simulink model "TEST_IPM_2_0"  (R2019b)
settings: configuration reference "Configuration" (kept outside this file)
PreLoadFcn:
  | RTWConfigurationCB('preloadfcn', bdroot);
values from neighbouring files (symbols this model uses):
  MParamFbase = 200.0    [TEST_IPM_LIB.sldd]
  MParamIbase = 360.0    [TEST_IPM_LIB.sldd]
  MParamLd = 8.0E-5    [TEST_IPM_LIB.sldd]
  MParamLq = 0.00028    [TEST_IPM_LIB.sldd]
  MParamRs = 0.014    [TEST_IPM_LIB.sldd]
  PWM_TPBRD_HALF = 5000.0    [TEST_IPM_LIB.sldd]
  Ts_10kHz = 0.0001    [TEST_IPM_LIB.sldd]
  Ts_1kHz = 0.001    [TEST_IPM_LIB.sldd]
undefined symbols (not defined in the file or in its folder): DiscIntNeverNeededParam, Down, GPTRIP1SEL, GPTRIP2SEL, TZ1, TZ2, Up
libraries: c280xlib x24, c2837xDlib x18, dsparch4 x11, c2802xlib x10, powerlib_meascontrol x9, dspstat3 x2, c2000lib x1, c2806xlib x1, idelinklib_common x1
(part 4 of 6)

== system TEST_IPM_2_0/INT/MAX5742/Subsystem3 ==
  function : TriggerPort  TriggerType=function-call  VariantControl=Variant
  Add1 : Sum
  Add3 : Sum  Commented=on
  Constant1 : Constant  Value=hex2dec('3000')  OutDataTypeStr=uint16  SampleTime=-1
  Constant6 : Constant  Commented=on  Value=hex2dec('3000')  OutDataTypeStr=uint16  SampleTime=-1
  Data Store Read : DataStoreRead  DataStoreName=Udc_FBK
  Data Store Read21 : DataStoreRead  Commented=on  DataStoreName=N_NOFILTER
  Gain1 : Gain  Commented=on  Gain=1/3000*4095
  Gain2 : Gain  Gain=1/80*4095
  SPI Transmit1 : c280xlib/SPI Transmit  SPISelect=SPI_B  ClockPolarity=Rising_edge  ClockPhase=No_delay  SPIModule=uint32(0)  Mode=Master  BusSpeed=uint32(1000000)  FirstBitToTransfer=Most significant bit (MSB)  ClockMode=0  BlockFunction=Write  EnableRegisterAddress=on  RegisterAddress=0  OutputDataType=int8  OutputDataLength=1  BlockingMode=off  DataBits=16  UseCustomSSPin=Provided by the SPI peripheral  ActiveLowSSPin=Active low  Pin=0
      settings: SourceProductName=Embedded Coder Support Package for Texas Instruments C2000 Processors  SourceProductBaseCode=TIC2000
  SPI Transmit3 : c280xlib/SPI Transmit  Commented=on  SPISelect=SPI_B  ClockPolarity=Rising_edge  ClockPhase=No_delay  SPIModule=uint32(0)  Mode=Master  BusSpeed=uint32(1000000)  FirstBitToTransfer=Most significant bit (MSB)  ClockMode=0  BlockFunction=Write  EnableRegisterAddress=on  RegisterAddress=0  OutputDataType=int8  OutputDataLength=1  BlockingMode=off  DataBits=16  UseCustomSSPin=Provided by the SPI peripheral  ActiveLowSSPin=Active low  Pin=0
      settings: SourceProductName=Embedded Coder Support Package for Texas Instruments C2000 Processors  SourceProductBaseCode=TIC2000
  Saturation1 : Saturate  UpperLimit=4095  LowerLimit=0  OutDataTypeStr=uint16
  Saturation3 : Saturate  Commented=on  UpperLimit=4095  LowerLimit=0  OutDataTypeStr=uint16
  Terminator1 : Terminator
  Terminator3 : Terminator  Commented=on
  wires:
  SPI Transmit3/1 -> Terminator3/1
  Constant6/1 -> Add3/2
  Gain1/1 -> Saturation3/1
  Saturation3/1 -> Add3/1
  Add3/1 -> SPI Transmit3/1
  Data Store Read21/1 -> Gain1/1
  Data Store Read/1 -> Gain2/1
  Add1/1 -> SPI Transmit1/1
  Saturation1/1 -> Add1/1
  Gain2/1 -> Saturation1/1
  Constant1/1 -> Add1/2
  SPI Transmit1/1 -> Terminator1/1

== system TEST_IPM_2_0/INT/MAX5742/Subsystem4 ==
  function : TriggerPort  TriggerType=function-call  VariantControl=Variant
  Add2 : Sum
  Constant1 : Constant  Value=hex2dec('0000')  OutDataTypeStr=uint16  SampleTime=-1
  Constant2 : Constant  Priority=102  Value=1024  OutDataTypeStr=Inherit: Inherit via back propagation  SampleTime=-1
  SPI Transmit : c280xlib/SPI Transmit  SPISelect=SPI_B  ClockPolarity=Rising_edge  ClockPhase=No_delay  SPIModule=uint32(0)  Mode=Master  BusSpeed=uint32(1000000)  FirstBitToTransfer=Most significant bit (MSB)  ClockMode=0  BlockFunction=Write  EnableRegisterAddress=on  RegisterAddress=0  OutputDataType=int8  OutputDataLength=1  BlockingMode=off  DataBits=16  UseCustomSSPin=Provided by the SPI peripheral  ActiveLowSSPin=Active low  Pin=0
      settings: SourceProductName=Embedded Coder Support Package for Texas Instruments C2000 Processors  SourceProductBaseCode=TIC2000
  Saturation : Saturate  UpperLimit=4095  LowerLimit=0  OutDataTypeStr=uint16
  Terminator : Terminator
  wires:
  Constant1/1 -> Add2/2
  SPI Transmit/1 -> Terminator/1
  Saturation/1 -> Add2/1
  Constant2/1 -> Saturation/1
  Add2/1 -> SPI Transmit/1

== system TEST_IPM_2_0/INT/MAX5742/Subsystem5 ==
  function : TriggerPort  TriggerType=function-call  VariantControl=Variant
  Add1 : Sum
  Constant1 : Constant  Priority=107  Value=2048  OutDataTypeStr=Inherit: Inherit via back propagation  SampleTime=-1
  Constant2 : Constant  Value=hex2dec('1000')  OutDataTypeStr=uint16  SampleTime=-1
  SPI Transmit1 : c280xlib/SPI Transmit  SPISelect=SPI_B  ClockPolarity=Rising_edge  ClockPhase=No_delay  SPIModule=uint32(0)  Mode=Master  BusSpeed=uint32(1000000)  FirstBitToTransfer=Most significant bit (MSB)  ClockMode=0  BlockFunction=Write  EnableRegisterAddress=on  RegisterAddress=0  OutputDataType=int8  OutputDataLength=1  BlockingMode=off  DataBits=16  UseCustomSSPin=Provided by the SPI peripheral  ActiveLowSSPin=Active low  Pin=0
      settings: SourceProductName=Embedded Coder Support Package for Texas Instruments C2000 Processors  SourceProductBaseCode=TIC2000
  Saturation1 : Saturate  UpperLimit=4095  LowerLimit=0  OutDataTypeStr=uint16
  Terminator1 : Terminator
  wires:
  Saturation1/1 -> Add1/1
  Add1/1 -> SPI Transmit1/1
  SPI Transmit1/1 -> Terminator1/1
  Constant2/1 -> Add1/2
  Constant1/1 -> Saturation1/1

== system TEST_IPM_2_0/INT/MAX5742/Subsystem6 ==
  function : TriggerPort  TriggerType=function-call  VariantControl=Variant
  Add4 : Sum
  Constant1 : Constant  Priority=112  Value=3072  OutDataTypeStr=Inherit: Inherit via back propagation  SampleTime=-1
  Constant5 : Constant  Value=hex2dec('2000')  OutDataTypeStr=uint16  SampleTime=-1
  SPI Transmit2 : c280xlib/SPI Transmit  SPISelect=SPI_B  ClockPolarity=Rising_edge  ClockPhase=No_delay  SPIModule=uint32(0)  Mode=Master  BusSpeed=uint32(1000000)  FirstBitToTransfer=Most significant bit (MSB)  ClockMode=0  BlockFunction=Write  EnableRegisterAddress=on  RegisterAddress=0  OutputDataType=int8  OutputDataLength=1  BlockingMode=off  DataBits=16  UseCustomSSPin=Provided by the SPI peripheral  ActiveLowSSPin=Active low  Pin=0
      settings: SourceProductName=Embedded Coder Support Package for Texas Instruments C2000 Processors  SourceProductBaseCode=TIC2000
  Saturation2 : Saturate  UpperLimit=4095  LowerLimit=0  OutDataTypeStr=uint16
  Terminator2 : Terminator
  wires:
  Constant5/1 -> Add4/2
  Saturation2/1 -> Add4/1
  Add4/1 -> SPI Transmit2/1
  SPI Transmit2/1 -> Terminator2/1
  Constant1/1 -> Saturation2/1

== system TEST_IPM_2_0/INT/MAX5742/Subsystem7 ==
  function : TriggerPort  TriggerType=function-call  VariantControl=Variant
  Add3 : Sum
  Constant6 : Constant  Value=hex2dec('3000')  OutDataTypeStr=uint16  SampleTime=-1
  Data Store Read : DataStoreRead  DataStoreName=UDCPROTECT
  SPI Transmit3 : c280xlib/SPI Transmit  SPISelect=SPI_B  ClockPolarity=Rising_edge  ClockPhase=No_delay  SPIModule=uint32(0)  Mode=Master  BusSpeed=uint32(1000000)  FirstBitToTransfer=Most significant bit (MSB)  ClockMode=0  BlockFunction=Write  EnableRegisterAddress=on  RegisterAddress=0  OutputDataType=int8  OutputDataLength=1  BlockingMode=off  DataBits=16  UseCustomSSPin=Provided by the SPI peripheral  ActiveLowSSPin=Active low  Pin=0
      settings: SourceProductName=Embedded Coder Support Package for Texas Instruments C2000 Processors  SourceProductBaseCode=TIC2000
  Saturation3 : Saturate  UpperLimit=4095  LowerLimit=0  OutDataTypeStr=uint16
  Terminator3 : Terminator
  wires:
  SPI Transmit3/1 -> Terminator3/1
  Constant6/1 -> Add3/2
  Data Store Read/1 -> Saturation3/1
  Saturation3/1 -> Add3/1
  Add3/1 -> SPI Transmit3/1

== system TEST_IPM_2_0/INT/Motor Control/Adjusting Mode ==
  Action Port : ActionPort  ActionPortLabel=case [ 0 ]:

== system TEST_IPM_2_0/INT/Motor Control/Clark Transformation ==
  U : Inport
  V : Inport  Port=2
  W : Inport  Port=3
  Add : Sum  Inputs=+--
  Add1 : Sum  Inputs=+-
  Gain : Gain  Gain=0.5
  Gain1 : Gain  Gain=0.5
  Gain2 : Gain  Gain=2/3
  Gain3 : Gain  Gain=2/3*0.86602540
  Alpha : Outport
  Beta : Outport  Port=2
  wires:
  V/1 -> Add1/1, Gain/1
  Gain/1 -> Add/2
  W/1 -> Add1/2, Gain1/1
  Gain1/1 -> Add/3
  U/1 -> Add/1
  Add/1 -> Gain2/1
  Gain2/1 -> Alpha/1
  Add1/1 -> Gain3/1
  Gain3/1 -> Beta/1

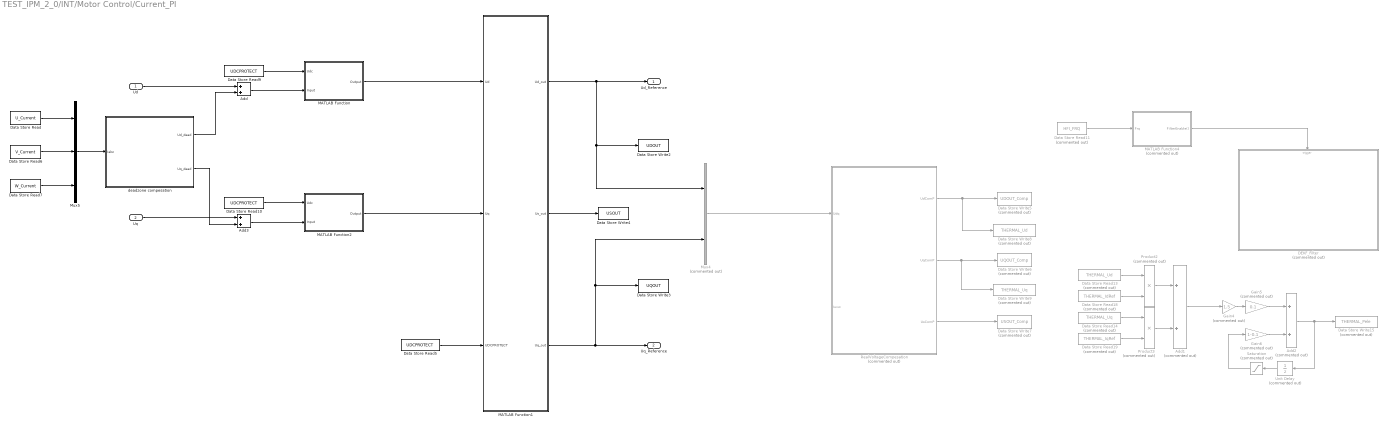
== system TEST_IPM_2_0/INT/Motor Control/Current_PI ==
  Ud : Inport
  Uq : Inport  Port=2
  Add : Sum
  Add1 : Sum  Commented=on
  Add2 : Sum  Commented=on
  Add3 : Sum
  DEKF_Filter : Subsystem  Commented=on  TreatAsAtomicUnit=on
  Data Store Read : DataStoreRead  DataStoreName=U_Current
  Data Store Read10 : DataStoreRead  DataStoreName=UDCPROTECT
  Data Store Read11 : DataStoreRead  Commented=on  DataStoreName=HFI_FRQ
  Data Store Read13 : DataStoreRead  Commented=on  DataStoreName=THERMAL_Ud
  Data Store Read14 : DataStoreRead  Commented=on  DataStoreName=THERMAL_Uq
  Data Store Read18 : DataStoreRead  Commented=on  DataStoreName=THERMAL_IdRef
  Data Store Read19 : DataStoreRead  Commented=on  DataStoreName=THERMAL_IqRef
  Data Store Read5 : DataStoreRead  DataStoreName=UDCPROTECT
  Data Store Read6 : DataStoreRead  DataStoreName=V_Current
  Data Store Read7 : DataStoreRead  DataStoreName=W_Current
  Data Store Read9 : DataStoreRead  DataStoreName=UDCPROTECT
  Data Store Write15 : DataStoreWrite  Commented=on  DataStoreName=THERMAL_Pele
  Data Store Write2 : DataStoreWrite  DataStoreName=UDOUT
  Data Store Write3 : DataStoreWrite  DataStoreName=UQOUT
  Data Store Write4 : DataStoreWrite  DataStoreName=USOUT
  Data Store Write5 : DataStoreWrite  Commented=on  DataStoreName=UDOUT_Comp
  Data Store Write6 : DataStoreWrite  Commented=on  DataStoreName=UQOUT_Comp
  Data Store Write7 : DataStoreWrite  Commented=on  DataStoreName=USOUT_Comp
  Data Store Write8 : DataStoreWrite  Commented=on  DataStoreName=THERMAL_Ud
  Data Store Write9 : DataStoreWrite  Commented=on  DataStoreName=THERMAL_Uq
  Gain4 : Gain  Commented=on  Gain=1.5
  Gain5 : Gain  Commented=on  Gain=0.1
  Gain6 : Gain  Commented=on  Gain=1-0.1
  MATLAB Function : MATLAB Function  TreatAsAtomicUnit=on
  MATLAB Function1 : MATLAB Function  TreatAsAtomicUnit=on
  MATLAB Function2 : MATLAB Function  TreatAsAtomicUnit=on
  MATLAB Function4 : MATLAB Function  Commented=on  TreatAsAtomicUnit=on
  Mux4 : Mux  Commented=on  Inputs=2
  Mux5 : Mux  Inputs=3
  Product2 : Product  Commented=on
  Product3 : Product  Commented=on
  "RealVoltageCompesation " : Subsystem  Commented=on  TreatAsAtomicUnit=on
  Saturation : Saturate  Commented=on  UpperLimit=100e3  LowerLimit=-100e3
  Unit Delay : UnitDelay  Commented=on  SampleTime=-1  HasFrameUpgradeWarning=on
  deadzone compesation : Subsystem
  Ud_Reference : Outport
  Uq_Reference : Outport  Port=2
  wires:
  MATLAB Function1/1(Ud_out) -> Ud_Reference/1, Data Store Write2/1, Mux4/1
  MATLAB Function1/3(Uq_out) -> Uq_Reference/1, Mux4/2, Data Store Write3/1
  MATLAB Function1/2(Us_out) -> Data Store Write4/1
  Data Store Read5/1 -> MATLAB Function1/3(UDCPROTECT)
  Mux4/1 -> "RealVoltageCompesation "/1(Udq)
  Data Store Read/1 -> Mux5/1
  Data Store Read6/1 -> Mux5/2
  Data Store Read7/1 -> Mux5/3
  Data Store Read9/1 -> MATLAB Function/1(Udc)
  Data Store Read10/1 -> MATLAB Function2/1(Udc)
  MATLAB Function/1(Output) -> MATLAB Function1/1(Ud)
  MATLAB Function2/1(Output) -> MATLAB Function1/2(Uq)
  "RealVoltageCompesation "/2(UqComP) -> Data Store Write9/1, Data Store Write6/1
  "RealVoltageCompesation "/3(UsComP) -> Data Store Write7/1
  "RealVoltageCompesation "/1(UdComP) -> Data Store Write8/1, Data Store Write5/1
  MATLAB Function4/1(FilterEnable()) -> DEKF_Filter/Trigger
  Data Store Read11/1 -> MATLAB Function4/1(Frq)
  Data Store Read13/1 -> Product2/1
  Data Store Read18/1 -> Product2/2
  Data Store Read14/1 -> Product3/1
  Data Store Read19/1 -> Product3/2
  Product2/1 -> Add1/1
  Product3/1 -> Add1/2
  Add1/1 -> Gain4/1
  Gain4/1 -> Gain5/1
  Add2/1 -> Unit Delay/1, Data Store Write15/1
  Unit Delay/1 -> Saturation/1
  Gain5/1 -> Add2/1
  Gain6/1 -> Add2/2
  Saturation/1 -> Gain6/1
  Add/1 -> MATLAB Function/2(Input)
  Ud/1 -> Add/1
  Add3/1 -> MATLAB Function2/2(Input)
  Uq/1 -> Add3/1
  deadzone compesation/1(Ud_dead) -> Add/2
  deadzone compesation/2(Uq_dead) -> Add3/2
  Mux5/1 -> deadzone compesation/1(Iabc)

== system TEST_IPM_2_0/INT/Motor Control/Error ==
  Action Port : ActionPort  ActionPortLabel=default:
  Constant : Constant  OutDataTypeStr=Inherit: Inherit via back propagation  SampleTime=-1
  Constant1 : Constant  Value=0  OutDataTypeStr=Inherit: Inherit via back propagation  SampleTime=-1
  Data Store Write1 : DataStoreWrite  DataStoreName=PROTECT
  Data Store Write2 : DataStoreWrite  DataStoreName=STOP
  wires:
  Constant/1 -> Data Store Write2/1
  Constant1/1 -> Data Store Write1/1

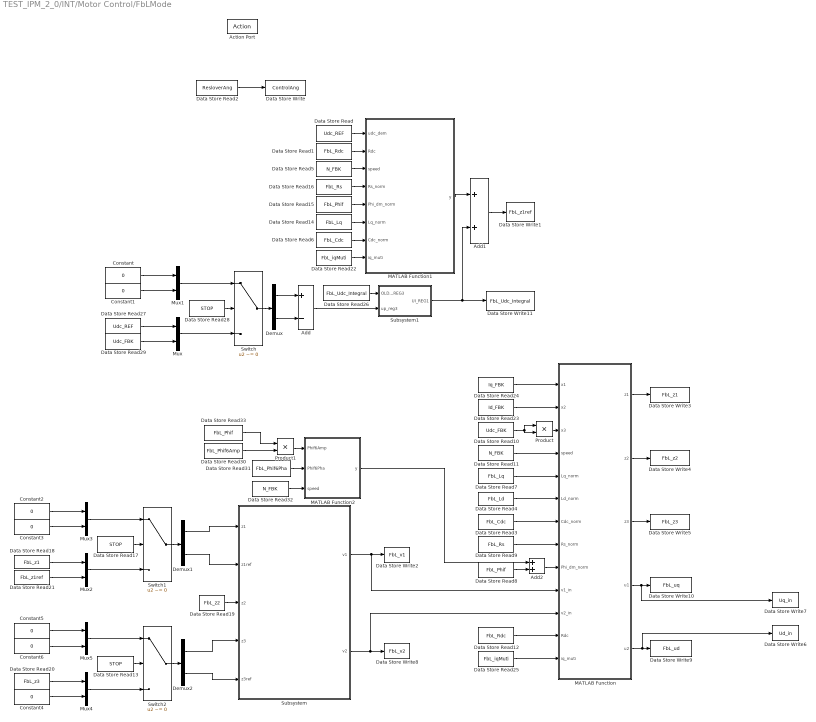
== system TEST_IPM_2_0/INT/Motor Control/FbLMode ==
  Action Port : ActionPort  ActionPortLabel=case [ 6 ]:
  Add : Sum  Inputs=+-
  Add1 : Sum
  Add2 : Sum
  Constant{,1..3,5..6} (6 alike) : Constant  Value=0  OutDataTypeStr=single  SampleTime=-1
  Constant4 : Constant  Value=0  OutDataTypeStr=single
  Data Store Read : DataStoreRead  DataStoreName=Udc_REF
  Data Store Read1 : DataStoreRead  DataStoreName=FbL_Rdc
  Data Store Read10 : DataStoreRead  DataStoreName=Udc_FBK
  Data Store Read11 : DataStoreRead  DataStoreName=N_FBK
  Data Store Read12 : DataStoreRead  DataStoreName=FbL_Rdc
  Data Store Read13 : DataStoreRead  DataStoreName=STOP
  Data Store Read14 : DataStoreRead  DataStoreName=FbL_Lq
  Data Store Read15 : DataStoreRead  DataStoreName=FbL_Phif
  Data Store Read16 : DataStoreRead  DataStoreName=FbL_Rs
  Data Store Read17 : DataStoreRead  DataStoreName=STOP
  Data Store Read18 : DataStoreRead  DataStoreName=FbL_z1
  Data Store Read19 : DataStoreRead  DataStoreName=FbL_z2
  Data Store Read2 : DataStoreRead  DataStoreName=ResloverAng
  Data Store Read20 : DataStoreRead  DataStoreName=FbL_z3
  Data Store Read21 : DataStoreRead  DataStoreName=FbL_z1ref
  Data Store Read22 : DataStoreRead  DataStoreName=FbL_iqMuti
  Data Store Read23 : DataStoreRead  DataStoreName=Id_FBK
  Data Store Read24 : DataStoreRead  DataStoreName=Iq_FBK
  Data Store Read25 : DataStoreRead  DataStoreName=FbL_iqMuti
  Data Store Read26 : DataStoreRead  DataStoreName=FbL_Udc_Integral
  Data Store Read27 : DataStoreRead  DataStoreName=Udc_REF
  Data Store Read28 : DataStoreRead  DataStoreName=STOP
  Data Store Read29 : DataStoreRead  DataStoreName=Udc_FBK
  Data Store Read3 : DataStoreRead  DataStoreName=FbL_Cdc
  Data Store Read30 : DataStoreRead  DataStoreName=FbL_Phif6Amp
  Data Store Read31 : DataStoreRead  DataStoreName=FbL_Phif6Pha
  Data Store Read32 : DataStoreRead  DataStoreName=N_FBK
  Data Store Read33 : DataStoreRead  DataStoreName=FbL_Phif
  Data Store Read4 : DataStoreRead  DataStoreName=FbL_Ld
  Data Store Read5 : DataStoreRead  DataStoreName=N_FBK
  Data Store Read6 : DataStoreRead  DataStoreName=FbL_Cdc
  Data Store Read7 : DataStoreRead  DataStoreName=FbL_Lq
  Data Store Read8 : DataStoreRead  DataStoreName=FbL_Phif
  Data Store Read9 : DataStoreRead  DataStoreName=FbL_Rs
  Data Store Write : DataStoreWrite  DataStoreName=ControlAng
  Data Store Write1 : DataStoreWrite  DataStoreName=FbL_z1ref
  Data Store Write10 : DataStoreWrite  DataStoreName=FbL_uq
  Data Store Write11 : DataStoreWrite  DataStoreName=FbL_Udc_Integral
  Data Store Write2 : DataStoreWrite  DataStoreName=FbL_v1
  Data Store Write3 : DataStoreWrite  DataStoreName=FbL_z1
  Data Store Write4 : DataStoreWrite  DataStoreName=FbL_z2
  Data Store Write5 : DataStoreWrite  DataStoreName=FbL_z3
  Data Store Write6 : DataStoreWrite  DataStoreName=Ud_in
  Data Store Write7 : DataStoreWrite  DataStoreName=Uq_in
  Data Store Write8 : DataStoreWrite  DataStoreName=FbL_v2
  Data Store Write9 : DataStoreWrite  DataStoreName=FbL_ud
  Demux : Demux  Outputs=2
  Demux1 : Demux  Outputs=2
  Demux2 : Demux  Outputs=2
  MATLAB Function : MATLAB Function  TreatAsAtomicUnit=on
  MATLAB Function1 : MATLAB Function  TreatAsAtomicUnit=on
  MATLAB Function2 : MATLAB Function  TreatAsAtomicUnit=on
  Mux{,1..5} (6 alike) : Mux  Inputs=2
  Product : Product
  Product1 : Product
  Subsystem : Subsystem
  Subsystem1 : Subsystem
  Switch : Switch  Criteria=u2 ~= 0
  Switch1 : Switch  Criteria=u2 ~= 0
  Switch2 : Switch  Criteria=u2 ~= 0
  wires:
  Data Store Read2/1 -> Data Store Write/1
  Data Store Read1/1 -> MATLAB Function1/2(Rdc)
  Data Store Read/1 -> MATLAB Function1/1(udc_dem)
  Data Store Read5/1 -> MATLAB Function1/3(speed)
  Data Store Read14/1 -> MATLAB Function1/6(Lq_norm)
  Data Store Read6/1 -> MATLAB Function1/7(Cdc_norm)
  Data Store Read16/1 -> MATLAB Function1/4(Rs_norm)
  Data Store Read15/1 -> MATLAB Function1/5(Phi_dm_norm)
  Subsystem1/1(UI_REG1) -> Data Store Write11/1, Add1/2
  Add/1 -> Subsystem1/2(up_reg3)
  MATLAB Function1/1(y) -> Add1/1
  Data Store Read19/1 -> Subsystem/3(z2)
  Add1/1 -> Data Store Write1/1
  Subsystem/1(v1) -> MATLAB Function/10(v1_in), Data Store Write2/1
  Subsystem/2(v2) -> Data Store Write8/1, MATLAB Function/11(v2_in)
  Data Store Read26/1 -> Subsystem1/1(OLD_UI_REG3)
  Data Store Read29/1 -> Mux/2
  Demux/2 -> Add/2
  Data Store Read27/1 -> Mux/1
  Demux/1 -> Add/1
  Constant/1 -> Mux1/1
  Constant1/1 -> Mux1/2
  Mux1/1 -> Switch/1
  Switch/1 -> Demux/1
  Data Store Read28/1 -> Switch/2
  Mux/1 -> Switch/3
  Data Store Read17/1 -> Switch1/2
  Constant3/1 -> Mux3/2
  Mux2/1 -> Switch1/3
  Constant2/1 -> Mux3/1
  Demux1/1 -> Subsystem/1(z1)
  Switch1/1 -> Demux1/1
  Demux1/2 -> Subsystem/2(z1ref)
  Mux3/1 -> Switch1/1
  Data Store Read18/1 -> Mux2/1
  Data Store Read21/1 -> Mux2/2
  Mux5/1 -> Switch2/1
  Switch2/1 -> Demux2/1
  Constant5/1 -> Mux5/1
  Mux4/1 -> Switch2/3
  Constant6/1 -> Mux5/2
  Data Store Read13/1 -> Switch2/2
  Data Store Read20/1 -> Mux4/1
  Constant4/1 -> Mux4/2
  Demux2/1 -> Subsystem/4(z3)
  Demux2/2 -> Subsystem/5(z3ref)
  Data Store Read7/1 -> MATLAB Function/5(Lq_norm)
  Data Store Read10/1 -> Product/2, Product/1
  Data Store Read3/1 -> MATLAB Function/7(Cdc_norm)
  MATLAB Function/5(u2) -> Data Store Write6/1, Data Store Write9/1
  Data Store Read24/1 -> MATLAB Function/1(x1)
  Data Store Read4/1 -> MATLAB Function/6(Ld_norm)
  MATLAB Function/1(z1) -> Data Store Write3/1
  Data Store Read9/1 -> MATLAB Function/8(Rs_norm)
  MATLAB Function/3(z3) -> Data Store Write5/1
  MATLAB Function/4(u1) -> Data Store Write7/1, Data Store Write10/1
  Data Store Read11/1 -> MATLAB Function/4(speed)
  MATLAB Function/2(z2) -> Data Store Write4/1
  Data Store Read12/1 -> MATLAB Function/12(Rdc)
  Product/1 -> MATLAB Function/3(x3)
  Data Store Read23/1 -> MATLAB Function/2(x2)
  Data Store Read22/1 -> MATLAB Function1/8(iq_muti)
  Data Store Read25/1 -> MATLAB Function/13(iq_muti)
  Data Store Read31/1 -> MATLAB Function2/2(Phif6Pha)
  Data Store Read32/1 -> MATLAB Function2/3(speed)
  Add2/1 -> MATLAB Function/9(Phi_dm_norm)
  Data Store Read8/1 -> Add2/2
  MATLAB Function2/1(y) -> Add2/1
  Product1/1 -> MATLAB Function2/1(Phif6Amp)
  Data Store Read30/1 -> Product1/2
  Data Store Read33/1 -> Product1/1

== system TEST_IPM_2_0/INT/Motor Control/IF ==
  Action Port : ActionPort  ActionPortLabel=case [ 2 ]:
  Data Store Read2 : DataStoreRead  DataStoreName=IF_F
  Data Store Read3 : DataStoreRead  DataStoreName=IF_F_Step
  Data Store Write : DataStoreWrite  DataStoreName=ControlAng
  Subsystem1 : Subsystem
  Subsystem2 : Subsystem
  wires:
  Data Store Read3/1 -> Subsystem1/2(Step)
  Data Store Read2/1 -> Subsystem1/1(TargetValue)
  Subsystem2/1(Ang) -> Data Store Write/1
  Subsystem1/1(RampOutput) -> Subsystem2/1(FRQ)

== system TEST_IPM_2_0/INT/Motor Control/Park Transformation ==
  Alpha : Inport
  Beta : Inport  Port=2
  theta : Inport  Port=3
  Add : Sum
  Add1 : Sum  Inputs=+-
  Product{,1..3} (4 alike) : Product
  Sin : Trigonometry  OutputSignalType=real
  Sin1 : Trigonometry  Operator=cos  OutputSignalType=real
  D : Outport
  Q : Outport  Port=2
  wires:
  Product/1 -> Add/1
  Sin/1 -> Product3/2, Product1/2
  Product1/1 -> Add/2
  Add1/1 -> Q/1
  Sin1/1 -> Product2/2, Product/2
  Product2/1 -> Add1/1
  Alpha/1 -> Product3/1, Product/1
  Beta/1 -> Product2/1, Product1/1
  Product3/1 -> Add1/2
  Add/1 -> D/1
  theta/1 -> Sin/1, Sin1/1

== system TEST_IPM_2_0/INT/Motor Control/SVPWM ==
  note: 由于矿车控制器ePWMxA是下管，B是上管，所以add变成了++
  Ud_Reference : Inport
  Uq_Reference : Inport  Port=2
  Angle : Inport  Port=3
  Add : Sum
  Constant1 : Constant  Value=PWM_TPBRD_HALF  OutDataTypeStr=single  SampleTime=-1
  Data Store Read3 : DataStoreRead  DataStoreName=ControlMode
  Data Store Read4 : DataStoreRead  DataStoreName=N_FBK
  Data Store Read5 : DataStoreRead  DataStoreName=Udc_FBK
  Demux : Demux  Outputs=2
  Divide : Product  Inputs=*/
  Gain : Gain  Gain=1/sqrt(3)
  Gain1 : Gain  Gain=PWM_TPBRD_HALF  OutDataTypeStr=single  ParamDataTypeStr=Inherit: Same as input
  Gain2 : Gain  Gain=4/60*2*pi*Ts_10kHz*1.5
  Inverse Park Transformation : Subsystem
  MATLAB Function : MATLAB Function  TreatAsAtomicUnit=on
  MATLAB Function1 : MATLAB Function  TreatAsAtomicUnit=on
  Mux : Mux  Inputs=2
  Mux1 : Mux  Inputs=3
  Saturation : Saturate  UpperLimit=370  LowerLimit=10
  Sum1 : Sum  Inputs=|-+  OutDataTypeStr=uint16
  COMPARE : Outport
  wires:
  Inverse Park Transformation/1(Alpha) -> MATLAB Function/1(alpha)
  Inverse Park Transformation/2(Beta) -> MATLAB Function/2(beta)
  Mux1/1 -> Gain1/1
  Sum1/1 -> COMPARE/1
  Gain1/1 -> Sum1/1
  Constant1/1 -> Sum1/2
  MATLAB Function/3(tc) -> Mux1/3
  MATLAB Function/2(tb) -> Mux1/2
  MATLAB Function/1(ta) -> Mux1/1
  Ud_Reference/1 -> Mux/1
  Uq_Reference/1 -> Mux/2
  Mux/1 -> Divide/1
  Saturation/1 -> Divide/2
  Gain/1 -> Saturation/1
  Demux/1 -> Inverse Park Transformation/1(D)
  Demux/2 -> Inverse Park Transformation/2(Q)
  Divide/1 -> Demux/1
  Data Store Read5/1 -> Gain/1
  Data Store Read4/1 -> Gain2/1
  Angle/1 -> Add/1
  Gain2/1 -> Add/2
  Add/1 -> MATLAB Function1/1(theta_in)
  Data Store Read3/1 -> MATLAB Function1/2(controlmode)
  MATLAB Function1/1(theta_out) -> Inverse Park Transformation/3(theta)

== system TEST_IPM_2_0/INT/Motor Control/SpeedMode ==
  Action Port : ActionPort  ActionPortLabel=case [ 4 ]:
  Constant3 : Constant  Value=MParamFbase*2*pi*MParamLq*1.5  OutDataTypeStr=Inherit: Inherit via back propagation  SampleTime=-1
  Constant4 : Constant  Value=MParamFbase*2*pi*MParamRs*1.5  OutDataTypeStr=Inherit: Inherit via back propagation  SampleTime=-1
  Constant5 : Constant  Value=MParamFbase*2*pi*MParamLq*1.5  OutDataTypeStr=Inherit: Inherit via back propagation  SampleTime=-1
  Constant6 : Constant  Value=MParamFbase*2*pi*MParamRs*1.5  OutDataTypeStr=Inherit: Inherit via back propagation  SampleTime=-1
  Data Store Read{,4..6} (4 alike) : DataStoreRead  DataStoreName=PI_Multi
  Data Store Read1 : DataStoreRead  Commented=on  DataStoreName=FLAG_MTPA
  Data Store Read2 : DataStoreRead  DataStoreName=ResloverAng
  Data Store Read3 : DataStoreRead  Commented=on  DataStoreName=Iq_REF
  Data Store Write : DataStoreWrite  DataStoreName=ControlAng
  Data Store Write3 : DataStoreWrite  DataStoreName=Id_Ki
  Data Store Write4 : DataStoreWrite  DataStoreName=Id_Kp
  Data Store Write5 : DataStoreWrite  DataStoreName=Iq_Ki
  Data Store Write6 : DataStoreWrite  DataStoreName=Iq_Kp
  Function-Call Subsystem : Subsystem  TreatAsAtomicUnit=on
  MATLAB Function : MATLAB Function  TreatAsAtomicUnit=on
  MATLAB Function1 : MATLAB Function  Commented=on  TreatAsAtomicUnit=on
  Product{,1..3} (4 alike) : Product
  wires:
  Data Store Read2/1 -> Data Store Write/1
  MATLAB Function/1(Speed_PI()) -> Function-Call Subsystem/Trigger
  Data Store Read3/1 -> MATLAB Function1/2(IqDem)
  Data Store Read1/1 -> MATLAB Function1/1(Flag_MTPA)
  MATLAB Function1/1(Id_REF) -> ?
  Product/1 -> Data Store Write4/1
  Data Store Read/1 -> Product/2
  Constant3/1 -> Product/1
  Constant4/1 -> Product1/1
  Data Store Read4/1 -> Product1/2
  Product1/1 -> Data Store Write3/1
  Product3/1 -> Data Store Write5/1
  Data Store Read6/1 -> Product3/2
  Constant6/1 -> Product3/1
  Constant5/1 -> Product2/1
  Data Store Read5/1 -> Product2/2
  Product2/1 -> Data Store Write6/1

== system TEST_IPM_2_0/INT/Motor Control/Stop  ==
  Action Port : ActionPort  ActionPortLabel=case [ 5 ]:
  Constant3 : Constant  OutDataTypeStr=Inherit: Inherit via back propagation  SampleTime=-1
  Constant4 : Constant  Value=0  OutDataTypeStr=Inherit: Inherit via back propagation  SampleTime=-1
  Data Store Write3 : DataStoreWrite  DataStoreName=PROTECT
  Data Store Write4 : DataStoreWrite  DataStoreName=STOP
  wires:
  Constant3/1 -> Data Store Write4/1
  Constant4/1 -> Data Store Write3/1

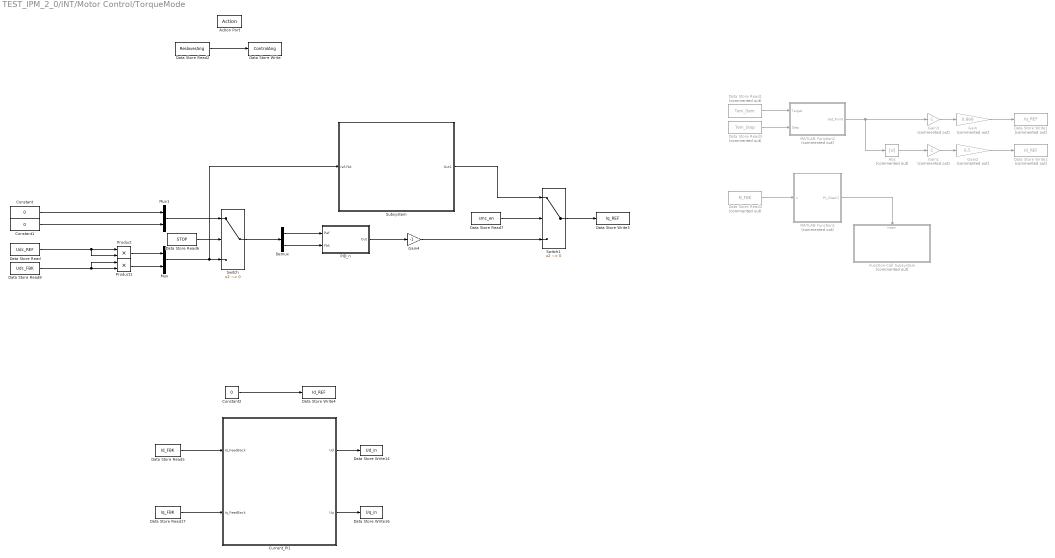
== system TEST_IPM_2_0/INT/Motor Control/TorqueMode ==
  Action Port : ActionPort  ActionPortLabel=case [ 3 ]:
  Abs : Abs  Commented=on
  Constant : Constant  Value=0  OutDataTypeStr=single  SampleTime=-1
  Constant1 : Constant  Value=0  OutDataTypeStr=single  SampleTime=-1
  Constant2 : Constant  Value=0  OutDataTypeStr=single
  Current_PI1 : Subsystem  TreatAsAtomicUnit=on
      settings: RTWSystemCode=Inline
  Data Store Read : DataStoreRead  DataStoreName=Udc_REF
  Data Store Read1 : DataStoreRead  Commented=on  DataStoreName=Tem_Dem
  Data Store Read17 : DataStoreRead  DataStoreName=Iq_FBK
  Data Store Read2 : DataStoreRead  DataStoreName=ResloverAng
  Data Store Read3 : DataStoreRead  Commented=on  DataStoreName=Tem_Step
  Data Store Read4 : DataStoreRead  Commented=on  DataStoreName=N_FBK
  Data Store Read5 : DataStoreRead  DataStoreName=Id_FBK
  Data Store Read6 : DataStoreRead  DataStoreName=STOP
  Data Store Read7 : DataStoreRead  DataStoreName=smc_en
  Data Store Read8 : DataStoreRead  DataStoreName=Udc_FBK
  Data Store Write : DataStoreWrite  DataStoreName=ControlAng
  Data Store Write1 : DataStoreWrite  Commented=on  DataStoreName=Iq_REF
  Data Store Write14 : DataStoreWrite  DataStoreName=Ud_in
  Data Store Write16 : DataStoreWrite  DataStoreName=Uq_in
  Data Store Write2 : DataStoreWrite  Commented=on  DataStoreName=Id_REF
  Data Store Write3 : DataStoreWrite  DataStoreName=Iq_REF
  Data Store Write4 : DataStoreWrite  DataStoreName=Id_REF
  Demux : Demux  Outputs=2
  Function-Call Subsystem : Subsystem  Commented=on  TreatAsAtomicUnit=on
  Gain : Gain  Commented=on  Gain=0.866
  Gain1 : Gain  Commented=on  Gain=-1  OutDataTypeStr=single
  Gain2 : Gain  Commented=on  Gain=0.5
  Gain3 : Gain  Commented=on  Gain=-1  OutDataTypeStr=single
  Gain4 : Gain  Gain=-1
  MATLAB Function1 : MATLAB Function  Commented=on  TreatAsAtomicUnit=on
  MATLAB Function2 : MATLAB Function  Commented=on  TreatAsAtomicUnit=on
  Mux : Mux  Inputs=2
  Mux1 : Mux  Inputs=2
  "PID_n " : Subsystem
  Product : Product
  Product1 : Product
  Subsystem : Subsystem
  Switch : Switch  Criteria=u2 ~= 0
  Switch1 : Switch  Criteria=u2 ~= 0
  wires:
  Data Store Read2/1 -> Data Store Write/1
  Data Store Read1/1 -> MATLAB Function2/1(Target)
  Data Store Read3/1 -> MATLAB Function2/2(Step)
  MATLAB Function2/1(Set_Point) -> Gain3/1, Abs/1
  Abs/1 -> Gain1/1
  Gain/1 -> Data Store Write1/1
  Gain1/1 -> Gain2/1
  Gain2/1 -> Data Store Write2/1
  Data Store Read4/1 -> MATLAB Function1/1(n)
  MATLAB Function1/1(PI_Clear()) -> Function-Call Subsystem/Trigger
  Gain3/1 -> Gain/1
  Demux/2 -> "PID_n "/2(Fbk)
  Mux/1 -> Subsystem/1(ref-fbk), Switch/3
  Mux1/1 -> Switch/1
  Constant/1 -> Mux1/1
  Switch/1 -> Demux/1
  Constant1/1 -> Mux1/2
  Demux/1 -> "PID_n "/1(Ref)
  Data Store Read6/1 -> Switch/2
  "PID_n "/1(Out) -> Gain4/1
  Constant2/1 -> Data Store Write4/1
  Current_PI1/2(Uq) -> Data Store Write16/1
  Current_PI1/1(Ud) -> Data Store Write14/1
  Data Store Read17/1 -> Current_PI1/2(Iq_FeedBack)
  Data Store Read5/1 -> Current_PI1/1(Id_FeedBack)
  Product/1 -> Mux/1
  Data Store Read/1 -> Product/2, Product/1
  Product1/1 -> Mux/2
  Data Store Read8/1 -> Product1/1, Product1/2
  Data Store Read7/1 -> Switch1/2
  Subsystem/1(Out1) -> Switch1/1
  Gain4/1 -> Switch1/3
  Switch1/1 -> Data Store Write3/1

== system TEST_IPM_2_0/INT/Motor Control/VF ==
  Action Port : ActionPort  ActionPortLabel=case [ 1 ]:
  Data Store Read : DataStoreRead  DataStoreName=VF_F
  Data Store Read2 : DataStoreRead  DataStoreName=VF_F_Step
  Data Store Write : DataStoreWrite  DataStoreName=ControlAng
  Subsystem1 : Subsystem
  Subsystem2 : Subsystem
  wires:
  Subsystem1/1(RampOutput) -> Subsystem2/1(FRQ)
  Subsystem2/1(Ang) -> Data Store Write/1
  Data Store Read/1 -> Subsystem1/1(TargetValue)
  Data Store Read2/1 -> Subsystem1/2(Step)

== system TEST_IPM_2_0/INT/Read Rotor Position/SpeedCal ==
  In1 : Inport
  function : TriggerPort  TriggerType=function-call  VariantControl=Variant
  "First Order Filter " : Subsystem
  MATLAB Function1 : MATLAB Function  TreatAsAtomicUnit=on
  Unit Delay : UnitDelay  SampleTime=-1  HasFrameUpgradeWarning=on
  Out1 : Outport
  wires:
  In1/1 -> Unit Delay/1, MATLAB Function1/1(theta)
  Unit Delay/1 -> MATLAB Function1/2(theta_old)
  MATLAB Function1/1(speed) -> "First Order Filter "/1(input)
  "First Order Filter "/1("output ") -> Out1/1

== system TEST_IPM_2_0/INT/ePWM/If Action Subsystem ==
  Action Port : ActionPort  ActionPortLabel=if(u1 == 1)
  Constant : Constant  Value=0  OutDataTypeStr=single  SampleTime=-1
  Data Store Write : DataStoreWrite  DataStoreName=N_Integral
  Data Store Write1 : DataStoreWrite  DataStoreName=Iq_Integral
  Data Store Write10 : DataStoreWrite  DataStoreName=FbL_z1_Integral
  Data Store Write12 : DataStoreWrite  DataStoreName=FbL_Udc_Integral
  Data Store Write2 : DataStoreWrite  DataStoreName=Id_Integral
  Data Store Write3 : DataStoreWrite  DataStoreName=Udc_Integral
  Data Store Write4 : DataStoreWrite  DataStoreName=smc_x1_integral
  Data Store Write5 : DataStoreWrite  DataStoreName=smc_e1_integral
  Data Store Write6 : DataStoreWrite  DataStoreName=smc_z1_integral
  Data Store Write7 : DataStoreWrite  DataStoreName=FbL_smc_integral
  Data Store Write9 : DataStoreWrite  DataStoreName=FbL_z3_Integral
  wires:
  Constant/1 -> Data Store Write3/1, Data Store Write10/1, Data Store Write7/1, Data Store Write6/1, Data Store Write5/1, Data Store Write4/1, Data Store Write12/1, Data Store Write9/1, Data Store Write1/1, Data Store Write2/1, Data Store Write/1

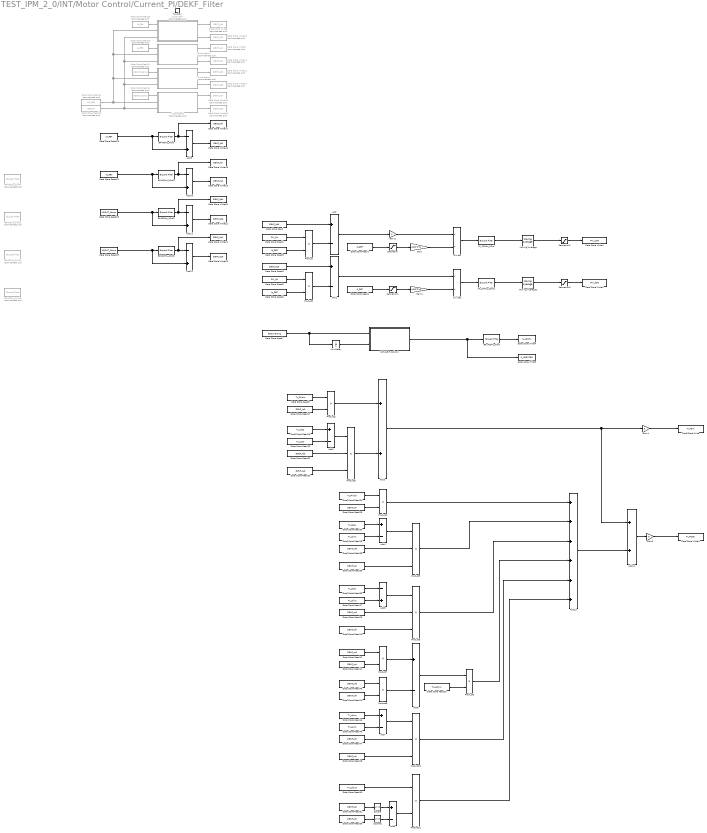
== system TEST_IPM_2_0/INT/Motor Control/Current_PI/DEKF_Filter ==
  function : TriggerPort  TriggerType=function-call  VariantControl=Variant  StatesWhenEnabling=reset
  Add{,1..2,4,6..8} (7 alike) : Sum  Inputs=+-
  Add{5,9..12} (5 alike) : Sum  Inputs=-+
  Add13 : Sum  Inputs=++++++
  Add14 : Sum
  Add3 : Sum
  BP400Hz_2Ord{1..4} (4 alike) : dsparch4/Biquad Filter  Tag=BlockMethodSubSystem  Commented=on  FilterSource=Dialog parameters  CoeffSource=Specify via dialog  FilterObject=BQF  IIRFiltStruct=Direct form II  BiQuadCoeffs=[1 0 -1 1 -1.92510858784585936 0.987511929907313402]  ScaleValues=[0.00624403504634327925;1]  IC=0  ICnum=0  ICden=0  a0Flag=Warning  optimizeScaleValues=on  ScaleValueMode=Specify via input port (g)  InputProcessing=Columns as channels (frame based)  roundingMode=Floor  overflowMode=off  scaleValueFracLength=14  denProdOutputFracLength=30  denAccumFracLength=30  secondMemoryFracLength=15
      settings: SourceProductName=DSP System Toolbox
  BP400Hz_4Ord{,1..3} (4 alike) : dsparch4/Biquad Filter  Tag=BlockMethodSubSystem  FilterSource=Dialog parameters  CoeffSource=Specify via dialog  FilterObject=BQF  IIRFiltStruct=Direct form II  BiQuadCoeffs=[1 0 -1 1 -1.93173306238314613 0.995528700328886185;1 0 -1 1 -1.93401211185528576 0.995605245274684303]  ScaleValues=[0.00313463184767947276;0.00313463184767947276;1]  IC=0  ICnum=0  ICden=0  a0Flag=Warning  optimizeScaleValues=on  ScaleValueMode=Specify via input port (g)  InputProcessing=Columns as channels (frame based)  roundingMode=Floor  overflowMode=off  scaleValueFracLength=14  denProdOutputFracLength=30  denAccumFracLength=30  secondMemoryFracLength=15
      settings: SourceProductName=DSP System Toolbox
  BP_400Hz_4Ord : dsparch4/Biquad Filter  Tag=BlockMethodSubSystem  FilterSource=Dialog parameters  CoeffSource=Specify via dialog  FilterObject=BQF  IIRFiltStruct=Direct form II  BiQuadCoeffs=[1 0 -1 1 -1.93173306238314613 0.995528700328886185;1 0 -1 1 -1.93401211185528576 0.995605245274684303]  ScaleValues=[0.00313463184767947276;0.00313463184767947276;1]  IC=0  ICnum=0  ICden=0  a0Flag=Warning  optimizeScaleValues=on  ScaleValueMode=Specify via input port (g)  InputProcessing=Columns as channels (frame based)  roundingMode=Floor  overflowMode=off  scaleValueFracLength=14  denProdOutputFracLength=30  denAccumFracLength=30  secondMemoryFracLength=15
      settings: SourceProductName=DSP System Toolbox
  Data Store Read : DataStoreRead  DataStoreName=DEKF_Ud0
  Data Store Read1 : DataStoreRead  DataStoreName=N_REF
  Data Store Read10 : DataStoreRead  DataStoreName=Tr_Lqap
  Data Store Read11 : DataStoreRead  Commented=on  DataStoreName=UDOUT_Comp
  Data Store Read12 : DataStoreRead  Commented=on  DataStoreName=HFI_FRQ
  Data Store Read13 : DataStoreRead  Commented=on  DataStoreName=DEKF_K
  Data Store Read14 : DataStoreRead  Commented=on  DataStoreName=UQOUT_Comp
  Data Store Read15 : DataStoreRead  DataStoreName=Tr_Lqinc
  Data Store Read16 : DataStoreRead  DataStoreName=Tr_Ldap
  Data Store Read17 : DataStoreRead  DataStoreName=Tr_Ldinc
  Data Store Read18 : DataStoreRead  DataStoreName=Id_FBK
  Data Store Read19 : DataStoreRead  DataStoreName=UDOUT_Comp
  Data Store Read2 : DataStoreRead  DataStoreName=Phi_Rs
  Data Store Read20 : DataStoreRead  DataStoreName=Tr_Ldqinc
  Data Store Read23 : DataStoreRead  DataStoreName=UQOUT_Comp
  Data Store Read24 : DataStoreRead  DataStoreName=Iq_FBK
  Data Store Read25 : DataStoreRead  Commented=on  DataStoreName=Id_FBK
  Data Store Read26 : DataStoreRead  Commented=on  DataStoreName=Iq_FBK
  Data Store Read{27,29,32,42} (4 alike) : DataStoreRead  DataStoreName=DEKF_Iq0
  Data Store Read{28,36,41,48,51} (5 alike) : DataStoreRead  DataStoreName=DEKF_Iqh
  Data Store Read3 : DataStoreRead  DataStoreName=DEKF_Uq0
  Data Store Read31 : DataStoreRead  DataStoreName=DEKF_Id0
  Data Store Read33 : DataStoreRead  DataStoreName=Tr_Ldap
  Data Store Read34 : DataStoreRead  DataStoreName=Tr_Phidm
  Data Store Read35 : DataStoreRead  DataStoreName=DEKF_Id0
  Data Store Read39 : DataStoreRead  DataStoreName=Tr_Lqap
  Data Store Read4 : DataStoreRead  DataStoreName=N_REF
  Data Store Read{40,44,47,50} (4 alike) : DataStoreRead  DataStoreName=DEKF_Idh
  Data Store Read43 : DataStoreRead  DataStoreName=DEKF_Id0
  Data Store Read45 : DataStoreRead  DataStoreName=Tr_Lqinc
  Data Store Read46 : DataStoreRead  DataStoreName=Tr_Ldinc
  Data Store Read49 : DataStoreRead  DataStoreName=Tr_Ldqinc
  Data Store Read5 : DataStoreRead  DataStoreName=Phi_Rs
  Data Store Read6 : DataStoreRead  DataStoreName=Iq_REF
  Data Store Read7 : DataStoreRead  DataStoreName=ResloverAng
  Data Store Read8 : DataStoreRead  DataStoreName=Tr_Phidm
  Data Store Read9 : DataStoreRead  DataStoreName=Id_REF
  Data Store Write : DataStoreWrite  DataStoreName=Tr_Tem
  Data Store Write1 : DataStoreWrite  DataStoreName=Phi_qOb
  Data Store Write10 : DataStoreWrite  Commented=on  DataStoreName=DEKF_Id0
  Data Store Write11 : DataStoreWrite  Commented=on  DataStoreName=DEKF_Iq0
  Data Store Write12 : DataStoreWrite  Commented=on  DataStoreName=DEKF_Udh
  Data Store Write13 : DataStoreWrite  Commented=on  DataStoreName=DEKF_Uqh
  Data Store Write14 : DataStoreWrite  Commented=on  DataStoreName=DEKF_Ud0
  Data Store Write15 : DataStoreWrite  Commented=on  DataStoreName=DEKF_Uq0
  Data Store Write16 : DataStoreWrite  DataStoreName=DEKF_Id0
  Data Store Write17 : DataStoreWrite  DataStoreName=DEKF_Idh
  Data Store Write18 : DataStoreWrite  DataStoreName=DEKF_Iqh
  Data Store Write19 : DataStoreWrite  DataStoreName=DEKF_Iq0
  Data Store Write2 : DataStoreWrite  DataStoreName=Phi_dOb
  Data Store Write20 : DataStoreWrite  DataStoreName=DEKF_Udh
  Data Store Write21 : DataStoreWrite  DataStoreName=DEKF_Uqh
  Data Store Write22 : DataStoreWrite  DataStoreName=DEKF_Ud0
  Data Store Write23 : DataStoreWrite  DataStoreName=DEKF_Uq0
  Data Store Write3 : DataStoreWrite  DataStoreName=Tr_Ttotal
  Data Store Write4 : DataStoreWrite  DataStoreName=N_400Hz
  Data Store Write5 : DataStoreWrite  DataStoreName=N_NOFILTER
  Data Store Write8 : DataStoreWrite  Commented=on  DataStoreName=DEKF_Idh
  Data Store Write9 : DataStoreWrite  Commented=on  DataStoreName=DEKF_Iqh
  Divide : Product  Inputs=*/
  Divide1 : Product  Inputs=*/
  Gain : Gain  Gain=4/60*2*pi
  Gain1 : Gain  Gain=4/60*2*pi
  Gain2 : Gain  Gain=-1
  Gain3 : Gain  Gain=6
  Gain4 : Gain  Gain=6
  LP_100Hz_2Ord : dsparch4/Biquad Filter  Tag=BlockMethodSubSystem  FilterSource=Dialog parameters  CoeffSource=Specify via dialog  FilterObject=BQF  IIRFiltStruct=Direct form II  BiQuadCoeffs=[1 2 1 1 -1.9111970674260732 0.914975834801433741]  ScaleValues=[0.000944691843840150748;1]  IC=0  ICnum=0  ICden=0  a0Flag=Warning  optimizeScaleValues=on  ScaleValueMode=Specify via input port (g)  InputProcessing=Columns as channels (frame based)  roundingMode=Floor  overflowMode=off  scaleValueFracLength=14  denProdOutputFracLength=30  denAccumFracLength=30  secondMemoryFracLength=15
      settings: SourceProductName=DSP System Toolbox
  LP_100Hz_2Ord1 : dsparch4/Biquad Filter  Tag=BlockMethodSubSystem  FilterSource=Dialog parameters  CoeffSource=Specify via dialog  FilterObject=BQF  IIRFiltStruct=Direct form II  BiQuadCoeffs=[1 2 1 1 -1.9111970674260732 0.914975834801433741]  ScaleValues=[0.000944691843840150748;1]  IC=0  ICnum=0  ICden=0  a0Flag=Warning  optimizeScaleValues=on  ScaleValueMode=Specify via input port (g)  InputProcessing=Columns as channels (frame based)  roundingMode=Floor  overflowMode=off  scaleValueFracLength=14  denProdOutputFracLength=30  denAccumFracLength=30  secondMemoryFracLength=15
      settings: SourceProductName=DSP System Toolbox
  MATLAB Function1 : MATLAB Function  TreatAsAtomicUnit=on
  Moving Average : dspstat3/Moving Average  Method=Sliding window  ForgettingFactorPort=off  SpecifyWindowLength=on  WindowLength=50  ForgettingFactor=0.9  SimulateUsing=Code generation
  Moving Average1 : dspstat3/Moving Average  Method=Sliding window  ForgettingFactorPort=off  SpecifyWindowLength=on  WindowLength=50  ForgettingFactor=0.9  SimulateUsing=Code generation
  Product{,1..2,4,7..9,11} (8 alike) : Product
  Product{3,5..6,10} (4 alike) : Product  Inputs=3
  Saturation : Saturate  UpperLimit=9000  LowerLimit=0.5
  Saturation1 : Saturate  UpperLimit=9000  LowerLimit=0.5
  Saturation2 : Saturate  UpperLimit=0.15  LowerLimit=-0.15
  Saturation3 : Saturate  UpperLimit=0.1  LowerLimit=-0.1
  Square : Math  Operator=square  SignedPower=off  OutputSignalType=real  OutDataTypeStr=single  SaturateOnIntegerOverflow=on
  Square1 : Math  Operator=square  SignedPower=off  OutputSignalType=real  OutDataTypeStr=single  SaturateOnIntegerOverflow=on
  Subsystem : Subsystem  Commented=on  TreatAsAtomicUnit=on
  Subsystem1 : Subsystem  Commented=on  TreatAsAtomicUnit=on
  Subsystem2 : Subsystem  Commented=on  TreatAsAtomicUnit=on
  Subsystem3 : Subsystem  Commented=on  TreatAsAtomicUnit=on
  Unit Delay : UnitDelay  SampleTime=-1  HasFrameUpgradeWarning=on
  wires:
  Data Store Read12/1 -> Subsystem/2("Frq "), Subsystem1/2("Frq "), Subsystem2/2("Frq "), Subsystem3/2("Frq ")
  Data Store Read26/1 -> Subsystem1/1("InputSignal ")
  Data Store Read25/1 -> Subsystem/1("InputSignal ")
  Subsystem2/3(BandStopSignal) -> Data Store Write14/1
  Data Store Read13/1 -> Subsystem/3(K), Subsystem1/3(K), Subsystem2/3(K), Subsystem3/3(K)
  Subsystem1/1(OutputSignal) -> Data Store Write9/1
  Data Store Read14/1 -> Subsystem3/1("InputSignal ")
  Subsystem/3(BandStopSignal) -> Data Store Write10/1
  Subsystem1/3(BandStopSignal) -> Data Store Write11/1
  Subsystem2/1(OutputSignal) -> Data Store Write12/1
  Subsystem/1(OutputSignal) -> Data Store Write8/1
  Subsystem3/1(OutputSignal) -> Data Store Write13/1
  Subsystem3/3(BandStopSignal) -> Data Store Write15/1
  Data Store Read11/1 -> Subsystem2/1("InputSignal ")
  BP400Hz_4Ord2/1 -> Data Store Write20/1, Add11/1
  Data Store Read23/1 -> BP400Hz_4Ord3/1, Add12/2
  BP400Hz_4Ord3/1 -> Data Store Write21/1, Add12/1
  Add12/1 -> Data Store Write23/1
  Data Store Read19/1 -> BP400Hz_4Ord2/1, Add11/2
  BP400Hz_4Ord1/1 -> Data Store Write18/1, Add10/1
  Add11/1 -> Data Store Write22/1
  Data Store Read18/1 -> BP400Hz_4Ord/1, Add9/2
  Data Store Read24/1 -> BP400Hz_4Ord1/1, Add10/2
  Add9/1 -> Data Store Write16/1
  Add10/1 -> Data Store Write19/1
  BP400Hz_4Ord/1 -> Data Store Write17/1, Add9/1
  Data Store Read2/1 -> Product/1
  Data Store Read/1 -> Add/1
  Data Store Read9/1 -> Product/2
  Product/1 -> Add/2
  Add/1 -> Gain2/1
  Data Store Read1/1 -> Saturation/1
  Saturation/1 -> Gain/1
  Gain/1 -> Divide/2
  Divide/1 -> LP_100Hz_2Ord/1
  Divide1/1 -> LP_100Hz_2Ord1/1
  Gain1/1 -> Divide1/2
  Saturation1/1 -> Gain1/1
  Data Store Read4/1 -> Saturation1/1
  Add1/1 -> Divide1/1
  Product1/1 -> Add1/2
  Data Store Read6/1 -> Product1/2
  Data Store Read3/1 -> Add1/1
  Data Store Read5/1 -> Product1/1
  Gain2/1 -> Divide/1
  LP_100Hz_2Ord/1 -> Moving Average/1
  LP_100Hz_2Ord1/1 -> Moving Average1/1
  BP_400Hz_4Ord/1 -> Data Store Write4/1
  Unit Delay/1 -> MATLAB Function1/2(theta_old)
  Data Store Read7/1 -> MATLAB Function1/1(theta), Unit Delay/1
  MATLAB Function1/1(speed) -> BP_400Hz_4Ord/1, Data Store Write5/1
  Saturation2/1 -> Data Store Write1/1
  Saturation3/1 -> Data Store Write2/1
  Moving Average/1 -> Saturation2/1
  Moving Average1/1 -> Saturation3/1
  Data Store Read8/1 -> Product2/1
  Data Store Read27/1 -> Product2/2
  Data Store Read16/1 -> Add2/1
  Data Store Read10/1 -> Add2/2
  Add2/1 -> Product3/1
  Data Store Read31/1 -> Product3/2
  Data Store Read32/1 -> Product3/3
  Product2/1 -> Add3/1
  Product3/1 -> Add3/2
  Add3/1 -> Add14/1, Gain4/1
  Data Store Read34/1 -> Product4/1
  Data Store Read28/1 -> Product4/2
  Data Store Read33/1 -> Add4/1
  Data Store Read15/1 -> Add4/2
  Add4/1 -> Product5/1
  Data Store Read35/1 -> Product5/2
  Data Store Read36/1 -> Product5/3
  Data Store Read39/1 -> Add5/1
  Data Store Read17/1 -> Add5/2
  Add5/1 -> Product6/1
  Data Store Read29/1 -> Product6/2
  Data Store Read40/1 -> Product6/3
  Data Store Read42/1 -> Product7/1
  Data Store Read41/1 -> Product7/2
  Data Store Read43/1 -> Product8/1
  Data Store Read44/1 -> Product8/2
  Product7/1 -> Add6/1
  Product8/1 -> Add6/2
  Add6/1 -> Product9/1
  Data Store Read20/1 -> Product9/2
  Data Store Read46/1 -> Add7/1
  Data Store Read45/1 -> Add7/2
  Add7/1 -> Product10/1
  Data Store Read47/1 -> Product10/2
  Data Store Read48/1 -> Product10/3
  Data Store Read49/1 -> Product11/1
  Add8/1 -> Product11/2
  Data Store Read51/1 -> Square/1
  Data Store Read50/1 -> Square1/1
  Square/1 -> Add8/1
  Square1/1 -> Add8/2
  Product4/1 -> Add13/1
  Product5/1 -> Add13/2
  Product6/1 -> Add13/3
  Product9/1 -> Add13/4
  Product10/1 -> Add13/5
  Product11/1 -> Add13/6
  Add13/1 -> Add14/2
  Add14/1 -> Gain3/1
  Gain3/1 -> Data Store Write3/1
  Gain4/1 -> Data Store Write/1

== system TEST_IPM_2_0/INT/Motor Control/Current_PI/RealVoltageCompesation  ==
  Udq : Inport
  Iuvw : Inport  Port=2
  Add : Sum  Inputs=+-
  Add1 : Sum  Inputs=+-
  Add2 : Sum  AccumDataTypeStr=single  OutDataTypeStr=single
  Clark Transformation : Subsystem
  Data Store Read : DataStoreRead  DataStoreName=K
  Data Store Read1 : DataStoreRead  DataStoreName=Udelta
  Data Store Read2 : DataStoreRead  DataStoreName=ControlAng
  Data Store Read3 : DataStoreRead  DataStoreName=N_REF
  Data Store Read4 : DataStoreRead  DataStoreName=DEKF_Udelay
  Delay : Delay
  Demux : Demux  Outputs=3
  Demux1 : Demux  Outputs=2
  Gain : Gain  Gain=4/60*2*pi*1e-4
  MATLAB Function : MATLAB Function  TreatAsAtomicUnit=on
  MATLAB Function1 : MATLAB Function  TreatAsAtomicUnit=on
  MATLAB Function2 : MATLAB Function  TreatAsAtomicUnit=on
  Park Transformation : Subsystem
  Park Transformation1 : Subsystem
  Product : Product
  Sqrt : Sqrt  OutputSignalType=real  OutDataTypeStr=single  IntermediateResultsDataTypeStr=single  SaturateOnIntegerOverflow=on
  Square : Math  Operator=square  SignedPower=off  OutputSignalType=real  OutDataTypeStr=single  SaturateOnIntegerOverflow=on
  Square1 : Math  Operator=square  SignedPower=off  OutputSignalType=real  OutDataTypeStr=single  SaturateOnIntegerOverflow=on
  UdComP : Outport
  UqComP : Outport  Port=2
  UsComP : Outport  Port=3
  wires:
  Udq/1 -> Delay/1
  Demux/1 -> MATLAB Function/1(I)
  Demux/2 -> MATLAB Function1/1(I)
  Demux/3 -> MATLAB Function2/1(I)
  Data Store Read/1 -> MATLAB Function2/2(K), MATLAB Function1/2(K), MATLAB Function/2(K)
  Data Store Read1/1 -> MATLAB Function/3(Udead), MATLAB Function1/3(Udead), MATLAB Function2/3(Udead)
  MATLAB Function/1(Uerror) -> Clark Transformation/1(U)
  MATLAB Function1/1(Uerror) -> Clark Transformation/2(V)
  MATLAB Function2/1(Uerror) -> Clark Transformation/3(W)
  Clark Transformation/1(Alpha) -> Park Transformation/1(Alpha)
  Clark Transformation/2(Beta) -> Park Transformation/2(Beta)
  Delay/1 -> Demux1/1
  Park Transformation/1(D) -> Add/2
  Park Transformation/2(Q) -> Add1/2
  Data Store Read3/1 -> Gain/1
  Demux1/1 -> Park Transformation1/1(Alpha)
  Demux1/2 -> Park Transformation1/2(Beta)
  Sqrt/1 -> UsComP/1
  Square1/1 -> Add2/2
  Add/1 -> Square/1, UdComP/1
  Square/1 -> Add2/1
  Add1/1 -> Square1/1, UqComP/1
  Add2/1 -> Sqrt/1
  Park Transformation1/1(D) -> Add/1
  Park Transformation1/2(Q) -> Add1/1
  Iuvw/1 -> Demux/1
  Data Store Read2/1 -> Park Transformation/3(theta)
  Product/1 -> Park Transformation1/3(theta)
  Gain/1 -> Product/1
  Data Store Read4/1 -> Product/2

== system TEST_IPM_2_0/INT/Motor Control/Current_PI/deadzone compesation ==
  Iabc : Inport
  Clark Transformation : Subsystem
  Data Store Read1 : DataStoreRead  DataStoreName=K
  Data Store Read2 : DataStoreRead  DataStoreName=Udelta
  Data Store Read3 : DataStoreRead  DataStoreName=ControlAng
  Demux : Demux  Outputs=3
  MATLAB Function3 : MATLAB Function  TreatAsAtomicUnit=on
  MATLAB Function5 : MATLAB Function  TreatAsAtomicUnit=on
  MATLAB Function6 : MATLAB Function  TreatAsAtomicUnit=on
  Park Transformation : Subsystem
  Ud_dead : Outport
  Uq_dead : Outport  Port=2
  wires:
  Park Transformation/2(Q) -> Uq_dead/1
  Clark Transformation/2(Beta) -> Park Transformation/2(Beta)
  Data Store Read1/1 -> MATLAB Function6/2(K), MATLAB Function5/2(K), MATLAB Function3/2(K)
  Clark Transformation/1(Alpha) -> Park Transformation/1(Alpha)
  Data Store Read2/1 -> MATLAB Function3/3(Udead), MATLAB Function5/3(Udead), MATLAB Function6/3(Udead)
  MATLAB Function5/1(Uerror) -> Clark Transformation/2(V)
  MATLAB Function6/1(Uerror) -> Clark Transformation/3(W)
  Demux/1 -> MATLAB Function3/1(I)
  MATLAB Function3/1(Uerror) -> Clark Transformation/1(U)
  Demux/2 -> MATLAB Function5/1(I)
  Demux/3 -> MATLAB Function6/1(I)
  Data Store Read3/1 -> Park Transformation/3(theta)
  Park Transformation/1(D) -> Ud_dead/1
  Iabc/1 -> Demux/1

== system TEST_IPM_2_0/INT/Motor Control/FbLMode/Subsystem ==
  z1 : Inport
  z1ref : Inport  Port=2
  z2 : Inport  Port=3
  z3 : Inport  Port=4
  z3ref : Inport  Port=5
  Add : Sum  Inputs=+++
  Data Store Read : DataStoreRead  DataStoreName=FbL_k2
  Gain : Gain  Gain=-1e-4  OutDataTypeStr=single
  "PID_z1 " : Subsystem  TreatAsAtomicUnit=on
  PID_z3 : Subsystem  TreatAsAtomicUnit=on
  Product : Product
  Subsystem : Subsystem
  v1 : Outport
  v2 : Outport  Port=2
  wires:
  z1/1 -> Subsystem/3(z1), "PID_z1 "/2(Fbk)
  Data Store Read/1 -> Gain/1
  Gain/1 -> Product/2
  z2/1 -> Subsystem/1(z2), Product/1
  z3/1 -> PID_z3/2(Fbk)
  z3ref/1 -> PID_z3/1(Ref)
  z1ref/1 -> Subsystem/2(z1ref), "PID_z1 "/1(Ref)
  Add/1 -> v1/1
  PID_z3/1(Out) -> v2/1
  "PID_z1 "/1(Out) -> Add/2
  Product/1 -> Add/3
  Subsystem/1(Out1) -> Add/1

== system TEST_IPM_2_0/INT/Motor Control/FbLMode/Subsystem1 ==
  OLD_UI_REG3 : Inport
  up_reg3 : Inport  Port=2
  Data Store Read1 : DataStoreRead  DataStoreName=FbL_k3
  Gain : Gain  Gain=Ts_10kHz
  Product1 : Product  OutDataTypeStr=Inherit: Same as first input
  Sum3 : Sum
  UI_REG1 : Outport
  wires:
  Data Store Read1/1 -> Gain/1
  Gain/1 -> Product1/1
  OLD_UI_REG3/1 -> Sum3/1
  Product1/1 -> Sum3/2
  up_reg3/1 -> Product1/2
  Sum3/1 -> UI_REG1/1

== system TEST_IPM_2_0/INT/Motor Control/IF/Subsystem1 ==
  TargetValue : Inport
  Step : Inport  Port=2
  MATLAB Function : MATLAB Function  TreatAsAtomicUnit=on
  Unit Delay : UnitDelay  SampleTime=-1  HasFrameUpgradeWarning=on
  RampOutput : Outport
  wires:
  TargetValue/1 -> MATLAB Function/1(Target)
  MATLAB Function/1(Output) -> RampOutput/1, Unit Delay/1
  Step/1 -> MATLAB Function/2(Step)
  Unit Delay/1 -> MATLAB Function/3(LastOutput)

== system TEST_IPM_2_0/INT/Motor Control/IF/Subsystem2 ==
  FRQ : Inport
  MATLAB Function : MATLAB Function  TreatAsAtomicUnit=on
  Unit Delay : UnitDelay  SampleTime=-1  HasFrameUpgradeWarning=on
  Ang : Outport
  wires:
  MATLAB Function/1(Ang) -> Ang/1, Unit Delay/1
  Unit Delay/1 -> MATLAB Function/2(LastAng)
  FRQ/1 -> MATLAB Function/1(FRQ)
